simulink model "SecRwLtStCaller"  (R2018b)
settings: Solver=FixedStepDiscrete  StartTime=0.0  StopTime=10.0  RelTol=1e-3
undefined symbols (not defined in the file): SecRwLtStArmScrnCtrl_1_Cal, SecRwLtStArmScrnHolderChk_1_Cal, SecRwLtStArmScrnIsPosChk_1_Cal, SecRwLtStArmScrnTrgtPosSelc_1_Cal, SecRwLtStBkReclnCtrl_1_Cal, SecRwLtStBkReclnHolderChk_1_Cal, SecRwLtStBkReclnIsPosChk_1_Cal, SecRwLtStBkReclnTrgtPosSelc_1_Cal, SecRwLtStChldLckChk_Cal, SecRwLtStFtrstCtrl_1_Cal, SecRwLtStFtrstHolderChk_1_Cal, SecRwLtStFtrstIsPosChk_1_Cal, SecRwLtStFtrstTrgtPosSelc_1_Cal, SecRwLtStFwdBkwdCtrl_1_Cal, SecRwLtStFwdBkwdHolderChk_1_Cal, SecRwLtStFwdBkwdIsPosChk_1_Cal, SecRwLtStFwdBkwdSpdCtrl_1_Cal, SecRwLtStFwdBkwdTrgtPosSelc_1_Cal, SecRwLtStHdrstFwdBkwdCtrl_1_Cal, SecRwLtStHdrstFwdBkwdHolderChk_1_Cal, SecRwLtStHdrstFwdBkwdIsPosChk_1_Cal, SecRwLtStHdrstFwdBkwdTrgtPosSelc_1_Cal, SecRwLtStHdrstUpwdDnwdCtrl_1_Cal, SecRwLtStHdrstUpwdDnwdHolderChk_1_Cal, SecRwLtStHdrstUpwdDnwdIsPosChk_1_Cal, SecRwLtStHdrstUpwdDnwdTrgtPosSelc_1_Cal, SecRwLtStHeightChk_Cal, SecRwLtStLgrstInwdOtwdCtrl_1_Cal, SecRwLtStLgrstInwdOtwdHolderChk_1_Cal, SecRwLtStLgrstInwdOtwdIsPosChk_1_Cal, SecRwLtStLgrstInwdOtwdTrgtPosSelc_1_Cal, SecRwLtStLgrstUpwdDnwdCtrl_1_Cal, SecRwLtStLgrstUpwdDnwdHolderChk_1_Cal, SecRwLtStLgrstUpwdDnwdIsPosChk_1_Cal, SecRwLtStLgrstUpwdDnwdTrgtPosSelc_1_Cal, SecRwLtStLtwdRtwdCtrl_1_Cal, SecRwLtStLtwdRtwdHolderChk_1_Cal, SecRwLtStLtwdRtwdIsPosChk_1_Cal, SecRwLtStLtwdRtwdTrgtPosSelc_1_Cal, SecRwLtStOccupyChk_Cal, SecRwLtStRclCmdSrvCal_1_Cal, SecRwLtStZeroCtrl_1_Cal, SecRwLtStZeroHolderChk_1_Cal, SecRwLtStZeroIsPosChk_1_Cal, SecRwLtStZeroTrgtPosSelc_1_Cal
settings Model: Creator=sn2xws  LastModifiedBy=sn2xws
settings Model: ModifiedHistory=|
  | 2024.5.6
  | 557 新增零重力电机
settings DataIOCC: SaveFormat=StructureWithTime
settings OptimizationCC: DefaultParameterBehavior=Inlined  EnhancedBackFolding=on  PassReuseOutputArgsAs=Individual arguments  ZeroExternalMemoryAtStartup=off  ZeroInternalMemoryAtStartup=off  OptimizeBlockOrder=speed  DifferentSizesBufferReuse=on  OptimizationCustomize=off
settings DebuggingCC: ParameterTunabilityLossMsg=error
settings SFSimCC: MATLABDynamicMemAlloc=off
settings RTWCC: SystemTargetFile=autosar.tlc  GenCodeOnly=on  TemplateMakefile=ert_default_tmf  Description=AUTOSAR  GenerateReport=on  IncludeHyperlinkInReport=on  LaunchReport=on  GenerateTraceInfo=on  GenerateTraceReport=on  GenerateTraceReportSl=on  GenerateTraceReportSf=on  GenerateTraceReportEml=on
settings CodeAppCC: ForceParamTrailComments=on  IgnoreCustomStorageClasses=off  OperatorAnnotations=on  SimulinkDataObjDesc=on  SFDataObjDesc=on  InsertBlockDesc=on
settings STFCustomTargetCC: TargetLangStandard=C99 (ISO)  MultiwordLength=256  ParMdlRefBuildCompliant=on  CompOptLevelCompliant=on  IncludeMdlTerminateFcn=off  CombineOutputUpdateFcns=on  SuppressErrorStatus=on  ERTCustomFileBanners=on  SupportNonFinite=off  SupportComplex=off  SupportContinuousTime=off  SupportNonInlinedSFcns=off  RemoveResetFunc=on  MATLABClassNameForMDSCustomization=Simulink.SoftwareTarget.ERTCustomization  AutosarCompliant=on  UseToolchainInfoCompliant=on  LookupTableObjectStructAxisOrder=2,1,3,4,...  LUTObjectStructOrderEvenSpacing=Size,Table,Breakpoints  SystemTargetFile=autosar.tlc
settings ERTTargetCC: TargetLangStandard=C99 (ISO)  ConcurrentExecutionCompliant=off  IncludeMdlTerminateFcn=off  SuppressErrorStatus=on  SupportNonFinite=off  SupportComplex=off  ModelStepFunctionPrototypeControlCompliant=off  CPPClassGenCompliant=off  AutosarCompliant=on  LookupTableObjectStructAxisOrder=2,1,3,4,...  LUTObjectStructOrderEvenSpacing=Size,Table,Breakpoints  InlinedParameterPlacement=NonHierarchical  ERTCustomFileTemplate=example_file_process.tlc  ERTFilePackagingFormat=Compact

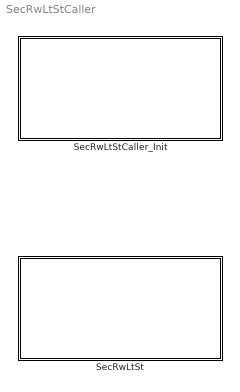
== system SecRwLtStCaller ==
  SecRwLtSt : Subsystem
  SecRwLtStCaller_Init : Subsystem

== system SecRwLtStCaller/SecRwLtSt ==
  SecRwLtSt_Cal_sys : Subsystem

== system SecRwLtStCaller/SecRwLtStCaller_Init ==
  Event Listener : EventListener  EventName=reset

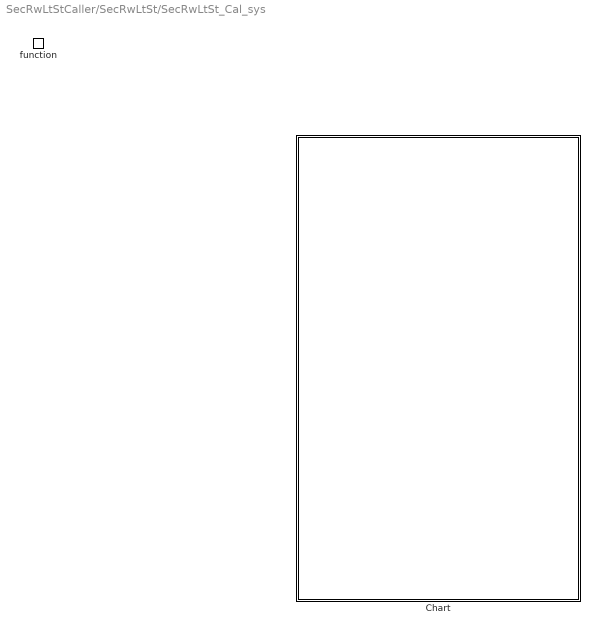
== system SecRwLtStCaller/SecRwLtSt/SecRwLtSt_Cal_sys ==
  function : TriggerPort  TriggerType=function-call  IsSimulinkFunction=on  FunctionName=SecRwLtSt_Cal  VariantControl=(inherit)
  Chart : Stateflow chart  TreatAsAtomicUnit=on

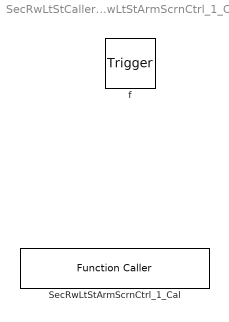
== system SecRwLtStCaller/SecRwLtSt/SecRwLtSt_Cal_sys/Chart/SecRwLtStArmScrnCtrl_1_Cal ==
  f : TriggerPort  TriggerType=function-call  VariantControl=(inherit)
      settings: CopyFcn=Stateflow.SLINSF.SimulinkMan.removeBlockPreDeleteFcn  PreDeleteFcn=Stateflow.SLINSF.SimulinkMan.unsafePredeleteFcn
  SecRwLtStArmScrnCtrl_1_Cal : FunctionCaller  FunctionPrototype=SecRwLtStArmScrnCtrl_1_Cal()

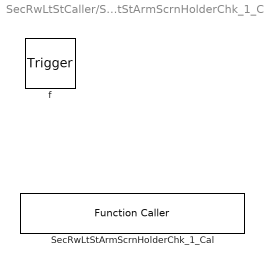
== system SecRwLtStCaller/SecRwLtSt/SecRwLtSt_Cal_sys/Chart/SecRwLtStArmScrnHolderChk_1_Cal ==
  f : TriggerPort  TriggerType=function-call  VariantControl=(inherit)
      settings: CopyFcn=Stateflow.SLINSF.SimulinkMan.removeBlockPreDeleteFcn  PreDeleteFcn=Stateflow.SLINSF.SimulinkMan.unsafePredeleteFcn
  SecRwLtStArmScrnHolderChk_1_Cal : FunctionCaller  FunctionPrototype=SecRwLtStArmScrnHolderChk_1_Cal()

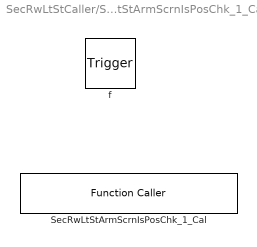
== system SecRwLtStCaller/SecRwLtSt/SecRwLtSt_Cal_sys/Chart/SecRwLtStArmScrnIsPosChk_1_Cal ==
  f : TriggerPort  TriggerType=function-call  VariantControl=(inherit)
      settings: CopyFcn=Stateflow.SLINSF.SimulinkMan.removeBlockPreDeleteFcn  PreDeleteFcn=Stateflow.SLINSF.SimulinkMan.unsafePredeleteFcn
  SecRwLtStArmScrnIsPosChk_1_Cal : FunctionCaller  FunctionPrototype=SecRwLtStArmScrnIsPosChk_1_Cal()

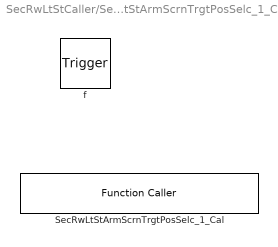
== system SecRwLtStCaller/SecRwLtSt/SecRwLtSt_Cal_sys/Chart/SecRwLtStArmScrnTrgtPosSelc_1_Cal ==
  f : TriggerPort  TriggerType=function-call  VariantControl=(inherit)
      settings: CopyFcn=Stateflow.SLINSF.SimulinkMan.removeBlockPreDeleteFcn  PreDeleteFcn=Stateflow.SLINSF.SimulinkMan.unsafePredeleteFcn
  SecRwLtStArmScrnTrgtPosSelc_1_Cal : FunctionCaller  FunctionPrototype=SecRwLtStArmScrnTrgtPosSelc_1_Cal()

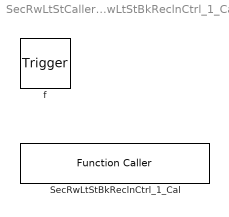
== system SecRwLtStCaller/SecRwLtSt/SecRwLtSt_Cal_sys/Chart/SecRwLtStBkReclnCtrl_1_Cal ==
  f : TriggerPort  TriggerType=function-call  VariantControl=(inherit)
      settings: CopyFcn=Stateflow.SLINSF.SimulinkMan.removeBlockPreDeleteFcn  PreDeleteFcn=Stateflow.SLINSF.SimulinkMan.unsafePredeleteFcn
  SecRwLtStBkReclnCtrl_1_Cal : FunctionCaller  FunctionPrototype=SecRwLtStBkReclnCtrl_1_Cal()

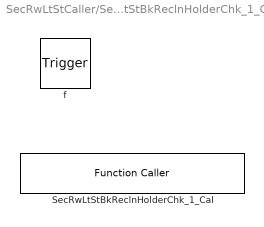
== system SecRwLtStCaller/SecRwLtSt/SecRwLtSt_Cal_sys/Chart/SecRwLtStBkReclnHolderChk_1_Cal ==
  f : TriggerPort  TriggerType=function-call  VariantControl=(inherit)
      settings: CopyFcn=Stateflow.SLINSF.SimulinkMan.removeBlockPreDeleteFcn  PreDeleteFcn=Stateflow.SLINSF.SimulinkMan.unsafePredeleteFcn
  SecRwLtStBkReclnHolderChk_1_Cal : FunctionCaller  FunctionPrototype=SecRwLtStBkReclnHolderChk_1_Cal()

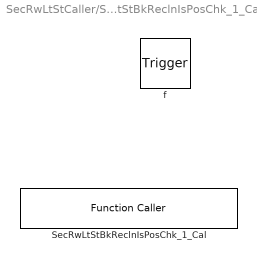
== system SecRwLtStCaller/SecRwLtSt/SecRwLtSt_Cal_sys/Chart/SecRwLtStBkReclnIsPosChk_1_Cal ==
  f : TriggerPort  TriggerType=function-call  VariantControl=(inherit)
      settings: CopyFcn=Stateflow.SLINSF.SimulinkMan.removeBlockPreDeleteFcn  PreDeleteFcn=Stateflow.SLINSF.SimulinkMan.unsafePredeleteFcn
  SecRwLtStBkReclnIsPosChk_1_Cal : FunctionCaller  FunctionPrototype=SecRwLtStBkReclnIsPosChk_1_Cal()

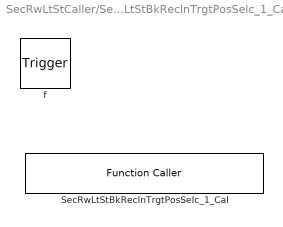
== system SecRwLtStCaller/SecRwLtSt/SecRwLtSt_Cal_sys/Chart/SecRwLtStBkReclnTrgtPosSelc_1_Cal ==
  f : TriggerPort  TriggerType=function-call  VariantControl=(inherit)
      settings: CopyFcn=Stateflow.SLINSF.SimulinkMan.removeBlockPreDeleteFcn  PreDeleteFcn=Stateflow.SLINSF.SimulinkMan.unsafePredeleteFcn
  SecRwLtStBkReclnTrgtPosSelc_1_Cal : FunctionCaller  FunctionPrototype=SecRwLtStBkReclnTrgtPosSelc_1_Cal()

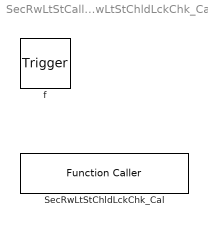
== system SecRwLtStCaller/SecRwLtSt/SecRwLtSt_Cal_sys/Chart/SecRwLtStChldLckChk_Cal ==
  f : TriggerPort  TriggerType=function-call  VariantControl=(inherit)
      settings: CopyFcn=Stateflow.SLINSF.SimulinkMan.removeBlockPreDeleteFcn  PreDeleteFcn=Stateflow.SLINSF.SimulinkMan.unsafePredeleteFcn
  SecRwLtStChldLckChk_Cal : FunctionCaller  FunctionPrototype=SecRwLtStChldLckChk_Cal()

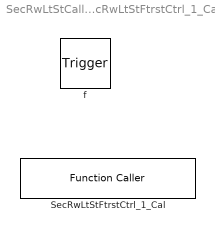
== system SecRwLtStCaller/SecRwLtSt/SecRwLtSt_Cal_sys/Chart/SecRwLtStFtrstCtrl_1_Cal ==
  f : TriggerPort  TriggerType=function-call  VariantControl=(inherit)
      settings: CopyFcn=Stateflow.SLINSF.SimulinkMan.removeBlockPreDeleteFcn  PreDeleteFcn=Stateflow.SLINSF.SimulinkMan.unsafePredeleteFcn
  SecRwLtStFtrstCtrl_1_Cal : FunctionCaller  FunctionPrototype=SecRwLtStFtrstCtrl_1_Cal()

== system SecRwLtStCaller/SecRwLtSt/SecRwLtSt_Cal_sys/Chart/SecRwLtStFtrstHolderChk_1_Cal ==
  f : TriggerPort  TriggerType=function-call  VariantControl=(inherit)
      settings: CopyFcn=Stateflow.SLINSF.SimulinkMan.removeBlockPreDeleteFcn  PreDeleteFcn=Stateflow.SLINSF.SimulinkMan.unsafePredeleteFcn
  SecRwLtStFtrstHolderChk_1_Cal : FunctionCaller  FunctionPrototype=SecRwLtStFtrstHolderChk_1_Cal()

== system SecRwLtStCaller/SecRwLtSt/SecRwLtSt_Cal_sys/Chart/SecRwLtStFtrstIsPosChk_1_Cal ==
  f : TriggerPort  TriggerType=function-call  VariantControl=(inherit)
      settings: CopyFcn=Stateflow.SLINSF.SimulinkMan.removeBlockPreDeleteFcn  PreDeleteFcn=Stateflow.SLINSF.SimulinkMan.unsafePredeleteFcn
  SecRwLtStFtrstIsPosChk_1_Cal : FunctionCaller  FunctionPrototype=SecRwLtStFtrstIsPosChk_1_Cal()

== system SecRwLtStCaller/SecRwLtSt/SecRwLtSt_Cal_sys/Chart/SecRwLtStFtrstTrgtPosSelc_1_Cal ==
  f : TriggerPort  TriggerType=function-call  VariantControl=(inherit)
      settings: CopyFcn=Stateflow.SLINSF.SimulinkMan.removeBlockPreDeleteFcn  PreDeleteFcn=Stateflow.SLINSF.SimulinkMan.unsafePredeleteFcn
  SecRwLtStFtrstTrgtPosSelc_1_Cal : FunctionCaller  FunctionPrototype=SecRwLtStFtrstTrgtPosSelc_1_Cal()

== system SecRwLtStCaller/SecRwLtSt/SecRwLtSt_Cal_sys/Chart/SecRwLtStFwdBkwdCtrl_1_Cal ==
  f : TriggerPort  TriggerType=function-call  VariantControl=(inherit)
      settings: CopyFcn=Stateflow.SLINSF.SimulinkMan.removeBlockPreDeleteFcn  PreDeleteFcn=Stateflow.SLINSF.SimulinkMan.unsafePredeleteFcn
  SecRwLtStFwdBkwdCtrl_1_Cal : FunctionCaller  FunctionPrototype=SecRwLtStFwdBkwdCtrl_1_Cal()

== system SecRwLtStCaller/SecRwLtSt/SecRwLtSt_Cal_sys/Chart/SecRwLtStFwdBkwdHolderChk_1_Cal ==
  f : TriggerPort  TriggerType=function-call  VariantControl=(inherit)
      settings: CopyFcn=Stateflow.SLINSF.SimulinkMan.removeBlockPreDeleteFcn  PreDeleteFcn=Stateflow.SLINSF.SimulinkMan.unsafePredeleteFcn
  SecRwLtStFwdBkwdHolderChk_1_Cal : FunctionCaller  FunctionPrototype=SecRwLtStFwdBkwdHolderChk_1_Cal()

== system SecRwLtStCaller/SecRwLtSt/SecRwLtSt_Cal_sys/Chart/SecRwLtStFwdBkwdIsPosChk_1_Cal ==
  f : TriggerPort  TriggerType=function-call  VariantControl=(inherit)
      settings: CopyFcn=Stateflow.SLINSF.SimulinkMan.removeBlockPreDeleteFcn  PreDeleteFcn=Stateflow.SLINSF.SimulinkMan.unsafePredeleteFcn
  SecRwLtStFwdBkwdIsPosChk_1_Cal : FunctionCaller  FunctionPrototype=SecRwLtStFwdBkwdIsPosChk_1_Cal()

== system SecRwLtStCaller/SecRwLtSt/SecRwLtSt_Cal_sys/Chart/SecRwLtStFwdBkwdSpdCtrl_1_Cal ==
  f : TriggerPort  TriggerType=function-call  VariantControl=(inherit)
      settings: CopyFcn=Stateflow.SLINSF.SimulinkMan.removeBlockPreDeleteFcn  PreDeleteFcn=Stateflow.SLINSF.SimulinkMan.unsafePredeleteFcn
  SecRwLtStFwdBkwdSpdCtrl_1_Cal : FunctionCaller  FunctionPrototype=SecRwLtStFwdBkwdSpdCtrl_1_Cal()

== system SecRwLtStCaller/SecRwLtSt/SecRwLtSt_Cal_sys/Chart/SecRwLtStFwdBkwdTrgtPosSelc_1_Cal ==
  f : TriggerPort  TriggerType=function-call  VariantControl=(inherit)
      settings: CopyFcn=Stateflow.SLINSF.SimulinkMan.removeBlockPreDeleteFcn  PreDeleteFcn=Stateflow.SLINSF.SimulinkMan.unsafePredeleteFcn
  SecRwLtStFwdBkwdTrgtPosSelc_1_Cal : FunctionCaller  FunctionPrototype=SecRwLtStFwdBkwdTrgtPosSelc_1_Cal()

== system SecRwLtStCaller/SecRwLtSt/SecRwLtSt_Cal_sys/Chart/SecRwLtStHdrstFwdBkwdCtrl_1_Cal ==
  f : TriggerPort  TriggerType=function-call  VariantControl=(inherit)
      settings: CopyFcn=Stateflow.SLINSF.SimulinkMan.removeBlockPreDeleteFcn  PreDeleteFcn=Stateflow.SLINSF.SimulinkMan.unsafePredeleteFcn
  SecRwLtStHdrstFwdBkwdCtrl_1_Cal : FunctionCaller  FunctionPrototype=SecRwLtStHdrstFwdBkwdCtrl_1_Cal()

== system SecRwLtStCaller/SecRwLtSt/SecRwLtSt_Cal_sys/Chart/SecRwLtStHdrstFwdBkwdHolderChk_1_Cal ==
  f : TriggerPort  TriggerType=function-call  VariantControl=(inherit)
      settings: CopyFcn=Stateflow.SLINSF.SimulinkMan.removeBlockPreDeleteFcn  PreDeleteFcn=Stateflow.SLINSF.SimulinkMan.unsafePredeleteFcn
  SecRwLtStHdrstFwdBkwdHolderChk_1_Cal : FunctionCaller  FunctionPrototype=SecRwLtStHdrstFwdBkwdHolderChk_1_Cal()

== system SecRwLtStCaller/SecRwLtSt/SecRwLtSt_Cal_sys/Chart/SecRwLtStHdrstFwdBkwdIsPosChk_1_Cal ==
  f : TriggerPort  TriggerType=function-call  VariantControl=(inherit)
      settings: CopyFcn=Stateflow.SLINSF.SimulinkMan.removeBlockPreDeleteFcn  PreDeleteFcn=Stateflow.SLINSF.SimulinkMan.unsafePredeleteFcn
  SecRwLtStHdrstFwdBkwdIsPosChk_1_Cal : FunctionCaller  FunctionPrototype=SecRwLtStHdrstFwdBkwdIsPosChk_1_Cal()

== system SecRwLtStCaller/SecRwLtSt/SecRwLtSt_Cal_sys/Chart/SecRwLtStHdrstFwdBkwdTrgtPosSelc_1_Cal ==
  f : TriggerPort  TriggerType=function-call  VariantControl=(inherit)
      settings: CopyFcn=Stateflow.SLINSF.SimulinkMan.removeBlockPreDeleteFcn  PreDeleteFcn=Stateflow.SLINSF.SimulinkMan.unsafePredeleteFcn
  SecRwLtStHdrstFwdBkwdTrgtPosSelc_1_Cal : FunctionCaller  FunctionPrototype=SecRwLtStHdrstFwdBkwdTrgtPosSelc_1_Cal()

== system SecRwLtStCaller/SecRwLtSt/SecRwLtSt_Cal_sys/Chart/SecRwLtStHdrstUpwdDnwdCtrl_1_Cal ==
  f : TriggerPort  TriggerType=function-call  VariantControl=(inherit)
      settings: CopyFcn=Stateflow.SLINSF.SimulinkMan.removeBlockPreDeleteFcn  PreDeleteFcn=Stateflow.SLINSF.SimulinkMan.unsafePredeleteFcn
  SecRwLtStHdrstUpwdDnwdCtrl_1_Cal : FunctionCaller  FunctionPrototype=SecRwLtStHdrstUpwdDnwdCtrl_1_Cal()

== system SecRwLtStCaller/SecRwLtSt/SecRwLtSt_Cal_sys/Chart/SecRwLtStHdrstUpwdDnwdHolderChk_1_Cal ==
  f : TriggerPort  TriggerType=function-call  VariantControl=(inherit)
      settings: CopyFcn=Stateflow.SLINSF.SimulinkMan.removeBlockPreDeleteFcn  PreDeleteFcn=Stateflow.SLINSF.SimulinkMan.unsafePredeleteFcn
  SecRwLtStHdrstUpwdDnwdHolderChk_1_Cal : FunctionCaller  FunctionPrototype=SecRwLtStHdrstUpwdDnwdHolderChk_1_Cal()

== system SecRwLtStCaller/SecRwLtSt/SecRwLtSt_Cal_sys/Chart/SecRwLtStHdrstUpwdDnwdIsPosChk_1_Cal ==
  f : TriggerPort  TriggerType=function-call  VariantControl=(inherit)
      settings: CopyFcn=Stateflow.SLINSF.SimulinkMan.removeBlockPreDeleteFcn  PreDeleteFcn=Stateflow.SLINSF.SimulinkMan.unsafePredeleteFcn
  SecRwLtStHdrstUpwdDnwdIsPosChk_1_Cal : FunctionCaller  FunctionPrototype=SecRwLtStHdrstUpwdDnwdIsPosChk_1_Cal()

== system SecRwLtStCaller/SecRwLtSt/SecRwLtSt_Cal_sys/Chart/SecRwLtStHdrstUpwdDnwdTrgtPosSelc_1_Cal ==
  f : TriggerPort  TriggerType=function-call  VariantControl=(inherit)
      settings: CopyFcn=Stateflow.SLINSF.SimulinkMan.removeBlockPreDeleteFcn  PreDeleteFcn=Stateflow.SLINSF.SimulinkMan.unsafePredeleteFcn
  SecRwLtStHdrstUpwdDnwdTrgtPosSelc_1_Cal : FunctionCaller  FunctionPrototype=SecRwLtStHdrstUpwdDnwdTrgtPosSelc_1_Cal()

== system SecRwLtStCaller/SecRwLtSt/SecRwLtSt_Cal_sys/Chart/SecRwLtStHeightChk_Cal ==
  f : TriggerPort  TriggerType=function-call  VariantControl=(inherit)
      settings: CopyFcn=Stateflow.SLINSF.SimulinkMan.removeBlockPreDeleteFcn  PreDeleteFcn=Stateflow.SLINSF.SimulinkMan.unsafePredeleteFcn
  SecRwLtStHeightChk_Cal : FunctionCaller  FunctionPrototype=SecRwLtStHeightChk_Cal()

== system SecRwLtStCaller/SecRwLtSt/SecRwLtSt_Cal_sys/Chart/SecRwLtStLgrstInwdOtwdCtrl_1_Cal ==
  f : TriggerPort  TriggerType=function-call  VariantControl=(inherit)
      settings: CopyFcn=Stateflow.SLINSF.SimulinkMan.removeBlockPreDeleteFcn  PreDeleteFcn=Stateflow.SLINSF.SimulinkMan.unsafePredeleteFcn
  SecRwLtStLgrstInwdOtwdCtrl_1_Cal : FunctionCaller  FunctionPrototype=SecRwLtStLgrstInwdOtwdCtrl_1_Cal()

== system SecRwLtStCaller/SecRwLtSt/SecRwLtSt_Cal_sys/Chart/SecRwLtStLgrstInwdOtwdHolderChk_1_Cal ==
  f : TriggerPort  TriggerType=function-call  VariantControl=(inherit)
      settings: CopyFcn=Stateflow.SLINSF.SimulinkMan.removeBlockPreDeleteFcn  PreDeleteFcn=Stateflow.SLINSF.SimulinkMan.unsafePredeleteFcn
  SecRwLtStLgrstInwdOtwdHolderChk_1_Cal : FunctionCaller  FunctionPrototype=SecRwLtStLgrstInwdOtwdHolderChk_1_Cal()

== system SecRwLtStCaller/SecRwLtSt/SecRwLtSt_Cal_sys/Chart/SecRwLtStLgrstInwdOtwdIsPosChk_1_Cal ==
  f : TriggerPort  TriggerType=function-call  VariantControl=(inherit)
      settings: CopyFcn=Stateflow.SLINSF.SimulinkMan.removeBlockPreDeleteFcn  PreDeleteFcn=Stateflow.SLINSF.SimulinkMan.unsafePredeleteFcn
  SecRwLtStLgrstInwdOtwdIsPosChk_1_Cal : FunctionCaller  FunctionPrototype=SecRwLtStLgrstInwdOtwdIsPosChk_1_Cal()

== system SecRwLtStCaller/SecRwLtSt/SecRwLtSt_Cal_sys/Chart/SecRwLtStLgrstInwdOtwdTrgtPosSelc_1_Cal ==
  f : TriggerPort  TriggerType=function-call  VariantControl=(inherit)
      settings: CopyFcn=Stateflow.SLINSF.SimulinkMan.removeBlockPreDeleteFcn  PreDeleteFcn=Stateflow.SLINSF.SimulinkMan.unsafePredeleteFcn
  SecRwLtStLgrstInwdOtwdTrgtPosSelc_1_Cal : FunctionCaller  FunctionPrototype=SecRwLtStLgrstInwdOtwdTrgtPosSelc_1_Cal()

== system SecRwLtStCaller/SecRwLtSt/SecRwLtSt_Cal_sys/Chart/SecRwLtStLgrstUpwdDnwdCtrl_1_Cal ==
  f : TriggerPort  TriggerType=function-call  VariantControl=(inherit)
      settings: CopyFcn=Stateflow.SLINSF.SimulinkMan.removeBlockPreDeleteFcn  PreDeleteFcn=Stateflow.SLINSF.SimulinkMan.unsafePredeleteFcn
  SecRwLtStLgrstUpwdDnwdCtrl_1_Cal : FunctionCaller  FunctionPrototype=SecRwLtStLgrstUpwdDnwdCtrl_1_Cal()

== system SecRwLtStCaller/SecRwLtSt/SecRwLtSt_Cal_sys/Chart/SecRwLtStLgrstUpwdDnwdHolderChk_1_Cal ==
  f : TriggerPort  TriggerType=function-call  VariantControl=(inherit)
      settings: CopyFcn=Stateflow.SLINSF.SimulinkMan.removeBlockPreDeleteFcn  PreDeleteFcn=Stateflow.SLINSF.SimulinkMan.unsafePredeleteFcn
  SecRwLtStLgrstUpwdDnwdHolderChk_1_Cal : FunctionCaller  FunctionPrototype=SecRwLtStLgrstUpwdDnwdHolderChk_1_Cal()

== system SecRwLtStCaller/SecRwLtSt/SecRwLtSt_Cal_sys/Chart/SecRwLtStLgrstUpwdDnwdIsPosChk_1_Cal ==
  f : TriggerPort  TriggerType=function-call  VariantControl=(inherit)
      settings: CopyFcn=Stateflow.SLINSF.SimulinkMan.removeBlockPreDeleteFcn  PreDeleteFcn=Stateflow.SLINSF.SimulinkMan.unsafePredeleteFcn
  SecRwLtStLgrstUpwdDnwdIsPosChk_1_Cal : FunctionCaller  FunctionPrototype=SecRwLtStLgrstUpwdDnwdIsPosChk_1_Cal()

== system SecRwLtStCaller/SecRwLtSt/SecRwLtSt_Cal_sys/Chart/SecRwLtStLgrstUpwdDnwdTrgtPosSelc_1_Cal ==
  f : TriggerPort  TriggerType=function-call  VariantControl=(inherit)
      settings: CopyFcn=Stateflow.SLINSF.SimulinkMan.removeBlockPreDeleteFcn  PreDeleteFcn=Stateflow.SLINSF.SimulinkMan.unsafePredeleteFcn
  SecRwLtStLgrstUpwdDnwdTrgtPosSelc_1_Cal : FunctionCaller  FunctionPrototype=SecRwLtStLgrstUpwdDnwdTrgtPosSelc_1_Cal()

== system SecRwLtStCaller/SecRwLtSt/SecRwLtSt_Cal_sys/Chart/SecRwLtStLtwdRtwdCtrl_1_Cal ==
  f : TriggerPort  TriggerType=function-call  VariantControl=(inherit)
      settings: CopyFcn=Stateflow.SLINSF.SimulinkMan.removeBlockPreDeleteFcn  PreDeleteFcn=Stateflow.SLINSF.SimulinkMan.unsafePredeleteFcn
  SecRwLtStLtwdRtwdCtrl_1_Cal : FunctionCaller  FunctionPrototype=SecRwLtStLtwdRtwdCtrl_1_Cal()

== system SecRwLtStCaller/SecRwLtSt/SecRwLtSt_Cal_sys/Chart/SecRwLtStLtwdRtwdHolderChk_1_Cal ==
  f : TriggerPort  TriggerType=function-call  VariantControl=(inherit)
      settings: CopyFcn=Stateflow.SLINSF.SimulinkMan.removeBlockPreDeleteFcn  PreDeleteFcn=Stateflow.SLINSF.SimulinkMan.unsafePredeleteFcn
  SecRwLtStLtwdRtwdHolderChk_1_Cal : FunctionCaller  FunctionPrototype=SecRwLtStLtwdRtwdHolderChk_1_Cal()

== system SecRwLtStCaller/SecRwLtSt/SecRwLtSt_Cal_sys/Chart/SecRwLtStLtwdRtwdIsPosChk_1_Cal ==
  f : TriggerPort  TriggerType=function-call  VariantControl=(inherit)
      settings: CopyFcn=Stateflow.SLINSF.SimulinkMan.removeBlockPreDeleteFcn  PreDeleteFcn=Stateflow.SLINSF.SimulinkMan.unsafePredeleteFcn
  SecRwLtStLtwdRtwdIsPosChk_1_Cal : FunctionCaller  FunctionPrototype=SecRwLtStLtwdRtwdIsPosChk_1_Cal()

== system SecRwLtStCaller/SecRwLtSt/SecRwLtSt_Cal_sys/Chart/SecRwLtStLtwdRtwdTrgtPosSelc_1_Cal ==
  f : TriggerPort  TriggerType=function-call  VariantControl=(inherit)
      settings: CopyFcn=Stateflow.SLINSF.SimulinkMan.removeBlockPreDeleteFcn  PreDeleteFcn=Stateflow.SLINSF.SimulinkMan.unsafePredeleteFcn
  SecRwLtStLtwdRtwdTrgtPosSelc_1_Cal : FunctionCaller  FunctionPrototype=SecRwLtStLtwdRtwdTrgtPosSelc_1_Cal()

== system SecRwLtStCaller/SecRwLtSt/SecRwLtSt_Cal_sys/Chart/SecRwLtStOccupyChk_Cal ==
  f : TriggerPort  TriggerType=function-call  VariantControl=(inherit)
      settings: CopyFcn=Stateflow.SLINSF.SimulinkMan.removeBlockPreDeleteFcn  PreDeleteFcn=Stateflow.SLINSF.SimulinkMan.unsafePredeleteFcn
  SecRwLtStOccupyChk_Cal : FunctionCaller  FunctionPrototype=SecRwLtStOccupyChk_Cal()

== system SecRwLtStCaller/SecRwLtSt/SecRwLtSt_Cal_sys/Chart/SecRwLtStRclCmdSrvCal_1_Cal ==
  f : TriggerPort  TriggerType=function-call  VariantControl=(inherit)
      settings: CopyFcn=Stateflow.SLINSF.SimulinkMan.removeBlockPreDeleteFcn  PreDeleteFcn=Stateflow.SLINSF.SimulinkMan.unsafePredeleteFcn
  SecRwLtStRclCmdSrvCal_1_Cal : FunctionCaller  FunctionPrototype=SecRwLtStRclCmdSrvCal_1_Cal()

== system SecRwLtStCaller/SecRwLtSt/SecRwLtSt_Cal_sys/Chart/SecRwLtStZeroCtrl_1_Cal ==
  note: Delete block
  f : TriggerPort  TriggerType=function-call  VariantControl=(inherit)
      settings: CopyFcn=Stateflow.SLINSF.SimulinkMan.removeBlockPreDeleteFcn  PreDeleteFcn=Stateflow.SLINSF.SimulinkMan.unsafePredeleteFcn
  SecRwLtStZeroCtrl_1_Cal : FunctionCaller  FunctionPrototype=SecRwLtStZeroCtrl_1_Cal()

== system SecRwLtStCaller/SecRwLtSt/SecRwLtSt_Cal_sys/Chart/SecRwLtStZeroHolderChk_1_Cal ==
  note: Delete block
  f : TriggerPort  TriggerType=function-call  VariantControl=(inherit)
      settings: CopyFcn=Stateflow.SLINSF.SimulinkMan.removeBlockPreDeleteFcn  PreDeleteFcn=Stateflow.SLINSF.SimulinkMan.unsafePredeleteFcn
  SecRwLtStZeroHolderChk_1_Cal : FunctionCaller  FunctionPrototype=SecRwLtStZeroHolderChk_1_Cal()

== system SecRwLtStCaller/SecRwLtSt/SecRwLtSt_Cal_sys/Chart/SecRwLtStZeroIsPosChk_1_Cal ==
  note: Delete block
  f : TriggerPort  TriggerType=function-call  VariantControl=(inherit)
      settings: CopyFcn=Stateflow.SLINSF.SimulinkMan.removeBlockPreDeleteFcn  PreDeleteFcn=Stateflow.SLINSF.SimulinkMan.unsafePredeleteFcn
  SecRwLtStZeroIsPosChk_1_Cal : FunctionCaller  FunctionPrototype=SecRwLtStZeroIsPosChk_1_Cal()

== system SecRwLtStCaller/SecRwLtSt/SecRwLtSt_Cal_sys/Chart/SecRwLtStZeroTrgtPosSelc_1_Cal ==
  note: Delete block
  f : TriggerPort  TriggerType=function-call  VariantControl=(inherit)
      settings: CopyFcn=Stateflow.SLINSF.SimulinkMan.removeBlockPreDeleteFcn  PreDeleteFcn=Stateflow.SLINSF.SimulinkMan.unsafePredeleteFcn
  SecRwLtStZeroTrgtPosSelc_1_Cal : FunctionCaller  FunctionPrototype=SecRwLtStZeroTrgtPosSelc_1_Cal()

== stateflow chart SecRwLtStCaller/SecRwLtSt/SecRwLtSt_Cal_sys/Chart ==
  state SecRwLtStChldLckChk_Cal [function]
  state SecRwLtStFtrstCtrl_1_Cal [function]
  state SecRwLtStBkReclnCtrl_1_Cal [function]
  state SecRwLtStArmScrnCtrl_1_Cal [function]
  state SecRwLtStFwdBkwdSpdCtrl_1_Cal [function]
  state SecRwLtStFtrstHolderChk_1_Cal [function]
  state SecRwLtStArmScrnHolderChk_1_Cal [function]
  state SecRwLtStBkReclnHolderChk_1_Cal [function]
  state SecRwLtStHeightChk_Cal [function]
  state SecRwLtStFtrstIsPosChk_1_Cal [function]
  state SecRwLtStArmScrnIsPosChk_1_Cal [function]
  state SecRwLtStBkReclnIsPosChk_1_Cal [function]
  state SecRwLtStOccupyChk_Cal [function]
  state SecRwLtStFtrstTrgtPosSelc_1_Cal [function]
  state SecRwLtStArmScrnTrgtPosSelc_1_Cal [function]
  state SecRwLtStBkReclnTrgtPosSelc_1_Cal [function]
  state SecRwLtStRclCmdSrvCal_1_Cal [function]
  state SecRwLtStFwdBkwdCtrl_1_Cal [function]
  state SecRwLtStHdrstFwdBkwdCtrl_1_Cal [function]
  state SecRwLtStHdrstUpwdDnwdCtrl_1_Cal [function]
  state SecRwLtStHdrstFwdBkwdHolderChk_1_Cal [function]
  state SecRwLtStFwdBkwdHolderChk_1_Cal [function]
  state SecRwLtStHdrstUpwdDnwdHolderChk_1_Cal [function]
  state SecRwLtStHdrstFwdBkwdIsPosChk_1_Cal [function]
  state SecRwLtStFwdBkwdIsPosChk_1_Cal [function]
  state SecRwLtStHdrstUpwdDnwdIsPosChk_1_Cal [function]
  state SecRwLtStHdrstFwdBkwdTrgtPosSelc_1_Cal [function]
  state SecRwLtStFwdBkwdTrgtPosSelc_1_Cal [function]
  state SecRwLtStHdrstUpwdDnwdTrgtPosSelc_1_Cal [function]
  state SecRwLtStLgrstInwdOtwdCtrl_1_Cal [function]
  state SecRwLtStLgrstUpwdDnwdCtrl_1_Cal [function]
  state SecRwLtStLtwdRtwdCtrl_1_Cal [function]
  state SecRwLtStLgrstInwdOtwdHolderChk_1_Cal [function]
  state SecRwLtStLgrstUpwdDnwdHolderChk_1_Cal [function]
  state SecRwLtStLtwdRtwdHolderChk_1_Cal [function]
  state SecRwLtStLgrstInwdOtwdIsPosChk_1_Cal [function]
  state SecRwLtStLgrstUpwdDnwdIsPosChk_1_Cal [function]
  state SecRwLtStLtwdRtwdIsPosChk_1_Cal [function]
  state SecRwLtStLgrstInwdOtwdTrgtPosSelc_1_Cal [function]
  state SecRwLtStLgrstUpwdDnwdTrgtPosSelc_1_Cal [function]
  state SecRwLtStLtwdRtwdTrgtPosSelc_1_Cal [function]
  state SecRwLtStZeroCtrl_1_Cal [function]
  state SecRwLtStZeroHolderChk_1_Cal [function]
  state SecRwLtStZeroIsPosChk_1_Cal [function]
  state SecRwLtStZeroTrgtPosSelc_1_Cal [function]
  (default) -> (junction 7)
  (junction 7) -> (junction 9) : {
      | SecRwLtStChldLckChk_Cal();
      | SecRwLtStHeightChk_Cal();
      | SecRwLtStOccupyChk_Cal();
      | SecRwLtStArmScrnTrgtPosSelc_1_Cal();
      | SecRwLtStArmScrnIsPosChk_1_Cal();
      | SecRwLtStArmScrnHolderChk_1_Cal();
      | SecRwLtStArmScrnCtrl_1_Cal();
      | SecRwLtStBkReclnTrgtPosSelc_1_Cal();
      | SecRwLtStBkReclnIsPosChk_1_Cal();
      | SecRwLtStBkReclnHolderChk_1_Cal();
      | SecRwLtStBkReclnCtrl_1_Cal();
      | SecRwLtStFtrstTrgtPosSelc_1_Cal();
      | SecRwLtStFtrstHolderChk_1_Cal();
      | SecRwLtStFtrstIsPosChk_1_Cal();
      | SecRwLtStFtrstCtrl_1_Cal();
      | SecRwLtStFwdBkwdTrgtPosSelc_1_Cal();
      | SecRwLtStFwdBkwdIsPosChk_1_Cal();
      | SecRwLtStFwdBkwdHolderChk_1_Cal();
      | SecRwLtStFwdBkwdCtrl_1_Cal();
      | SecRwLtStFwdBkwdSpdCtrl_1_Cal();
      | SecRwLtStHdrstFwdBkwdTrgtPosSelc_1_Cal();
      | SecRwLtStHdrstFwdBkwdIsPosChk_1_Cal();
      | SecRwLtStHdrstFwdBkwdHolderChk_1_Cal();
      | SecRwLtStHdrstFwdBkwdCtrl_1_Cal();
      | SecRwLtStHdrstUpwdDnwdTrgtPosSelc_1_Cal();
      | SecRwLtStHdrstUpwdDnwdIsPosChk_1_Cal();
      | SecRwLtStHdrstUpwdDnwdHolderChk_1_Cal();
      | SecRwLtStHdrstUpwdDnwdCtrl_1_Cal();
      | SecRwLtStLgrstInwdOtwdTrgtPosSelc_1_Cal();
      | SecRwLtStLgrstInwdOtwdIsPosChk_1_Cal();
      | SecRwLtStLgrstInwdOtwdHolderChk_1_Cal();
      | SecRwLtStLgrstInwdOtwdCtrl_1_Cal();
      | SecRwLtStLgrstUpwdDnwdTrgtPosSelc_1_Cal();
      | SecRwLtStLgrstUpwdDnwdIsPosChk_1_Cal();
      | SecRwLtStLgrstUpwdDnwdHolderChk_1_Cal();
      | SecRwLtStLgrstUpwdDnwdCtrl_1_Cal();
      | SecRwLtStLtwdRtwdTrgtPosSelc_1_Cal();
      | SecRwLtStLtwdRtwdIsPosChk_1_Cal();
      | SecRwLtStLtwdRtwdHolderChk_1_Cal();
      | SecRwLtStLtwdRtwdCtrl_1_Cal();
      | SecRwLtStZeroTrgtPosSelc_1_Cal();
      | SecRwLtStZeroIsPosChk_1_Cal();
      | SecRwLtStZeroHolderChk_1_Cal();
      | SecRwLtStZeroCtrl_1_Cal();
      | SecRwLtStRclCmdSrvCal_1_Cal();
      | }
